simulink model "AFS_Model"  (R2021a)
settings: Solver=FixedStepDiscrete  StartTime=0.0  StopTime=1  FixedStep=0.2  RelTol=1e-3
libraries: simulink x25
settings Model: DataDictionary=AFLS.sldd  Creator=Prajakta  LastModifiedBy=hp
settings DataIOCC: ExternalInput=[t,Longi_Distance,Lat_Distance,Lux,Wheel_Angle,Speed]  LoadExternalInput=on
settings OptimizationCC: DefaultParameterBehavior=Inlined  EnhancedBackFolding=on  PassReuseOutputArgsAs=Individual arguments  ZeroExternalMemoryAtStartup=off  ZeroInternalMemoryAtStartup=off  OptimizeBlockOrder=speed  DifferentSizesBufferReuse=on  OptimizationCustomize=off  EfficientTunableParamExpr=on
settings DebuggingCC: ParameterTunabilityLossMsg=error
settings SFSimCC: MATLABDynamicMemAlloc=off
settings RTWCC: SystemTargetFile=ert.tlc  GenCodeOnly=on  TemplateMakefile=ert_default_tmf  GenerateReport=on  IncludeHyperlinkInReport=on  LaunchReport=on  GenerateTraceInfo=on  GenerateWebview=on
settings CodeAppCC: ForceParamTrailComments=on  IgnoreCustomStorageClasses=off  OperatorAnnotations=on  SimulinkDataObjDesc=on  SFDataObjDesc=on  InsertBlockDesc=on
settings ERTTargetCC: TargetLangStandard=C99 (ISO)  GenerateSampleERTMain=on  InlinedParameterPlacement=NonHierarchical  ERTCustomFileTemplate=example_file_process.tlc

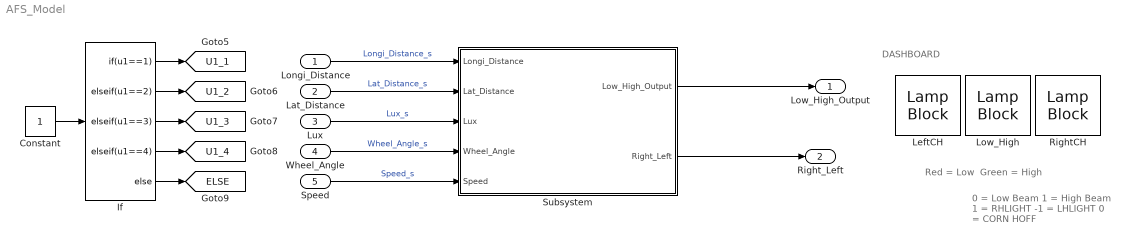
== system AFS_Model ==
  note: Green = High
  note: Red = Low
  note: 0 = Low Beam
      | 1 = High Beam
      | 1 = RHLIGHT
      | -1 = LHLIGHT
      | 0 = CORN HOFF
  note: DASHBOARD
  Longi_Distance : Inport
  Lat_Distance : Inport  Port=2
  Lux : Inport  Port=3
  Wheel_Angle : Inport  Port=4
  Speed : Inport  Port=5
  Constant : Constant
  If : If  IfExpression=u1==1  ElseIfExpressions=u1==2, u1==3,u1==4
  LeftCH : LampBlock
  Low_High : LampBlock
  RightCH : LampBlock
  Subsystem : Subsystem
  Low_High_Output : Outport
  Right_Left : Outport  Port=2
  tag scope: ELSE=global, U1_1=global, U1_2=global, U1_3=global, U1_4=global
  wires:
  If/1 -> [U1_1]
  If/2 -> [U1_2]
  If/3 -> [U1_3]
  If/4 -> [U1_4]
  If/5 -> [ELSE]
  Longi_Distance/1 -> Subsystem/1(Longi_Distance)  "Longi_Distance_s"
  Lat_Distance/1 -> Subsystem/2(Lat_Distance)  "Lat_Distance_s"
  Lux/1 -> Subsystem/3(Lux)  "Lux_s"
  Wheel_Angle/1 -> Subsystem/4(Wheel_Angle)  "Wheel_Angle_s"
  Speed/1 -> Subsystem/5(Speed)  "Speed_s"
  Subsystem/1(Low_High_Output) -> Low_High_Output/1
  Subsystem/2(Right_Left) -> Right_Left/1
  Constant/1 -> If/1

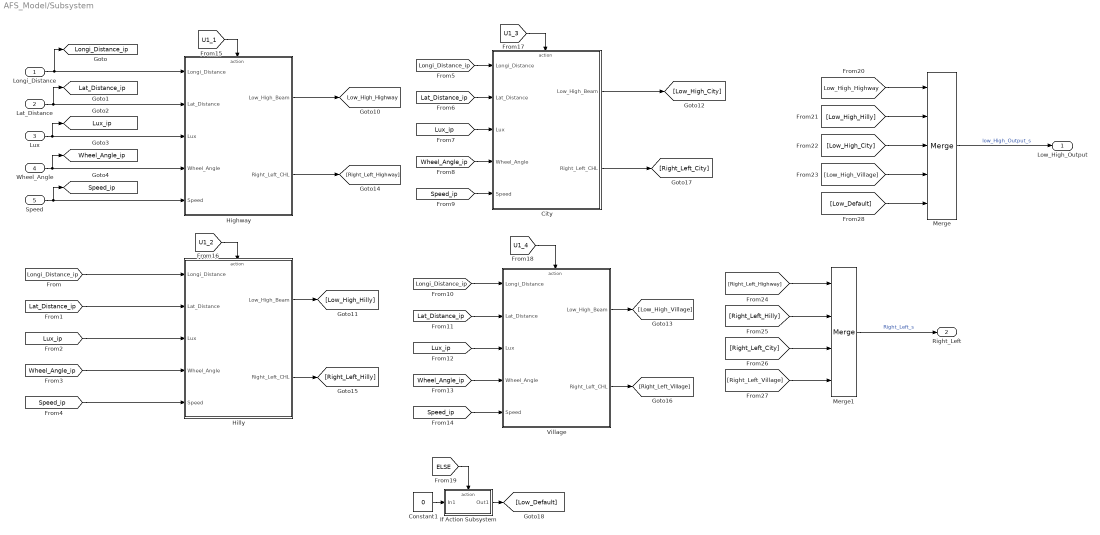
== system AFS_Model/Subsystem ==
  Longi_Distance : Inport
  Lat_Distance : Inport  Port=2
  Lux : Inport  Port=3
  Wheel_Angle : Inport  Port=4
  Speed : Inport  Port=5
  City : Subsystem  TreatAsAtomicUnit=on
  Constant1 : Constant  Value=0  OutDataTypeStr=int8
  Highway : Subsystem  TreatAsAtomicUnit=on
  Hilly : Subsystem  TreatAsAtomicUnit=on
  If Action Subsystem : Subsystem  TreatAsAtomicUnit=on
  Merge : Merge  Inputs=5
  Merge1 : Merge  Inputs=4
  Village : Subsystem  TreatAsAtomicUnit=on
  Low_High_Output : Outport
  Right_Left : Outport  Port=2  OutDataTypeStr=int8
  tag scope: Lat_Distance_ip=global, Longi_Distance_ip=global, Low_High_Highway=global, Lux_ip=global, Speed_ip=global, Wheel_Angle_ip=global
  wires:
  [ELSE] -> If Action Subsystem/Action
  [Wheel_Angle_ip] -> Hilly/4(Wheel_Angle)
  Longi_Distance/1 -> Highway/1(Longi_Distance), [Longi_Distance_ip]
  [Longi_Distance_ip] -> City/1(Longi_Distance)
  [Speed_ip] -> Hilly/5(Speed)
  [Low_High_Highway] -> Merge/1
  Lat_Distance/1 -> Highway/2(Lat_Distance), [Lat_Distance_ip]
  [Lux_ip] -> Hilly/3(Lux)
  [U1_2] -> Hilly/Action
  [U1_3] -> City/Action
  Wheel_Angle/1 -> Highway/4(Wheel_Angle), [Wheel_Angle_ip]
  [Low_Default] -> Merge/5
  City/2(Right_Left_CHL) -> [Right_Left_City]
  [Longi_Distance_ip] -> Hilly/1(Longi_Distance)
  Speed/1 -> Highway/5(Speed), [Speed_ip]
  [Wheel_Angle_ip] -> Village/4(Wheel_Angle)
  [Lat_Distance_ip] -> Hilly/2(Lat_Distance)
  [Lat_Distance_ip] -> City/2(Lat_Distance)
  Merge1/1 -> Right_Left/1  "Right_Left_s"
  Highway/2(Right_Left_CHL) -> [Right_Left_Highway]
  [Wheel_Angle_ip] -> City/4(Wheel_Angle)
  Highway/1(Low_High_Beam) -> [Low_High_Highway]
  Constant1/1 -> If Action Subsystem/1(In1)
  [U1_1] -> Highway/Action
  [Speed_ip] -> City/5(Speed)
  [Right_Left_Highway] -> Merge1/1
  [Longi_Distance_ip] -> Village/1(Longi_Distance)
  [U1_4] -> Village/Action
  Hilly/1(Low_High_Beam) -> [Low_High_Hilly]
  Lux/1 -> Highway/3(Lux), [Lux_ip]
  Hilly/2(Right_Left_CHL) -> [Right_Left_Hilly]
  Village/2(Right_Left_CHL) -> [Right_Left_Village]
  [Right_Left_Village] -> Merge1/4
  [Lux_ip] -> City/3(Lux)
  [Lat_Distance_ip] -> Village/2(Lat_Distance)
  [Right_Left_City] -> Merge1/3
  Village/1(Low_High_Beam) -> [Low_High_Village]
  [Speed_ip] -> Village/5(Speed)
  If Action Subsystem/1(Out1) -> [Low_Default]
  [Low_High_City] -> Merge/3
  [Lux_ip] -> Village/3(Lux)
  [Low_High_Village] -> Merge/4
  Merge/1 -> Low_High_Output/1  "low_High_Output_s"
  [Right_Left_Hilly] -> Merge1/2
  [Low_High_Hilly] -> Merge/2
  City/1(Low_High_Beam) -> [Low_High_City]

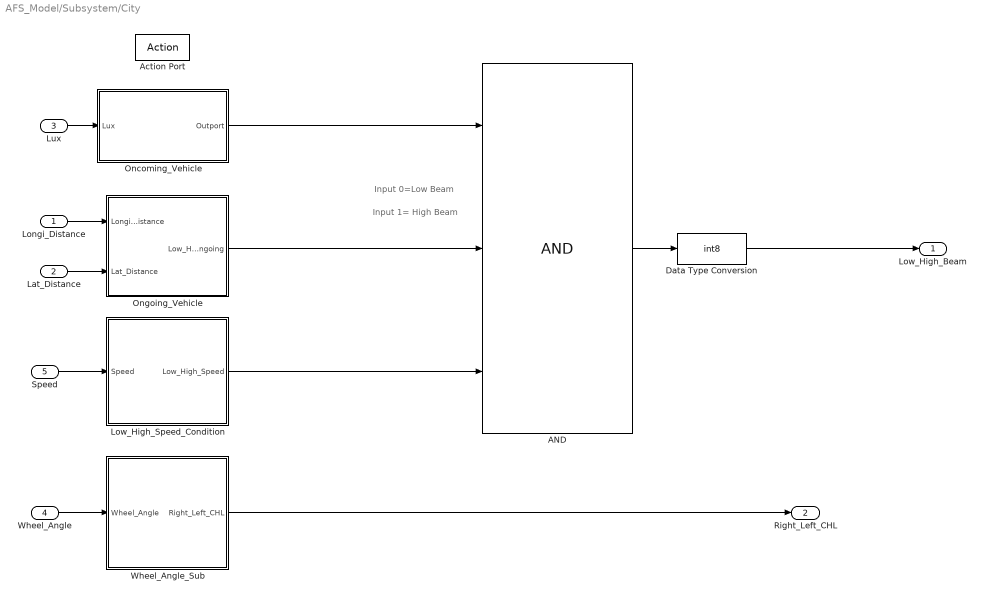
== system AFS_Model/Subsystem/City ==
  note: Input 1= High Beam
  note: Input 0=Low Beam
  Longi_Distance : Inport
  Lat_Distance : Inport  Port=2
  Lux : Inport  Port=3
  Wheel_Angle : Inport  Port=4
  Speed : Inport  Port=5
  Action Port : ActionPort  ActionPortLabel=elseif( u1==3)
  AND : Logic  Inputs=3  AllPortsSameDT=off  OutDataTypeStr=boolean
  Data Type Conversion : DataTypeConversion  OutDataTypeStr=int8
  Low_High_Speed_Condition : Subsystem
  Oncoming_Vehicle : Subsystem
  Ongoing_Vehicle : Subsystem
  Wheel_Angle_Sub : Subsystem
  Low_High_Beam : Outport
  Right_Left_CHL : Outport  Port=2
  wires:
  Longi_Distance/1 -> Ongoing_Vehicle/1(Longi_Distance)
  Lat_Distance/1 -> Ongoing_Vehicle/2(Lat_Distance)
  Lux/1 -> Oncoming_Vehicle/1(Lux)
  Oncoming_Vehicle/1(Outport) -> AND/1
  AND/1 -> Data Type Conversion/1
  Ongoing_Vehicle/1(Low_High_Ongoing) -> AND/2
  Data Type Conversion/1 -> Low_High_Beam/1
  Wheel_Angle/1 -> Wheel_Angle_Sub/1(Wheel_Angle)
  Wheel_Angle_Sub/1(Right_Left_CHL) -> Right_Left_CHL/1
  Low_High_Speed_Condition/1(Low_High_Speed) -> AND/3
  Speed/1 -> Low_High_Speed_Condition/1(Speed)

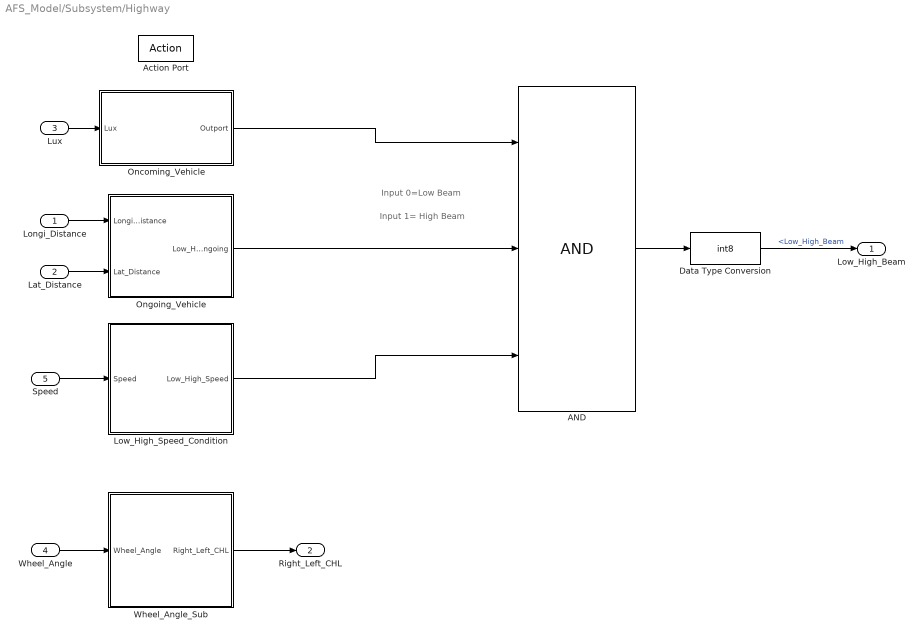
== system AFS_Model/Subsystem/Highway ==
  note: Input 1= High Beam
  note: Input 0=Low Beam
  Longi_Distance : Inport
  Lat_Distance : Inport  Port=2
  Lux : Inport  Port=3
  Wheel_Angle : Inport  Port=4
  Speed : Inport  Port=5
  Action Port : ActionPort  ActionPortLabel=if(u1==1)
  AND : Logic  Inputs=3  AllPortsSameDT=off  OutDataTypeStr=boolean
  Data Type Conversion : DataTypeConversion  OutDataTypeStr=int8
  Low_High_Speed_Condition : Subsystem
  Oncoming_Vehicle : Subsystem
  Ongoing_Vehicle : Subsystem
  Wheel_Angle_Sub : Subsystem
  Low_High_Beam : Outport
  Right_Left_CHL : Outport  Port=2
  wires:
  Longi_Distance/1 -> Ongoing_Vehicle/1(Longi_Distance)
  Lat_Distance/1 -> Ongoing_Vehicle/2(Lat_Distance)
  Lux/1 -> Oncoming_Vehicle/1(Lux)
  Oncoming_Vehicle/1(Outport) -> AND/1
  AND/1 -> Data Type Conversion/1
  Ongoing_Vehicle/1(Low_High_Ongoing) -> AND/2
  Data Type Conversion/1 -> Low_High_Beam/1  "<Low_High_Beam"
  Wheel_Angle/1 -> Wheel_Angle_Sub/1(Wheel_Angle)
  Wheel_Angle_Sub/1(Right_Left_CHL) -> Right_Left_CHL/1
  Low_High_Speed_Condition/1(Low_High_Speed) -> AND/3
  Speed/1 -> Low_High_Speed_Condition/1(Speed)

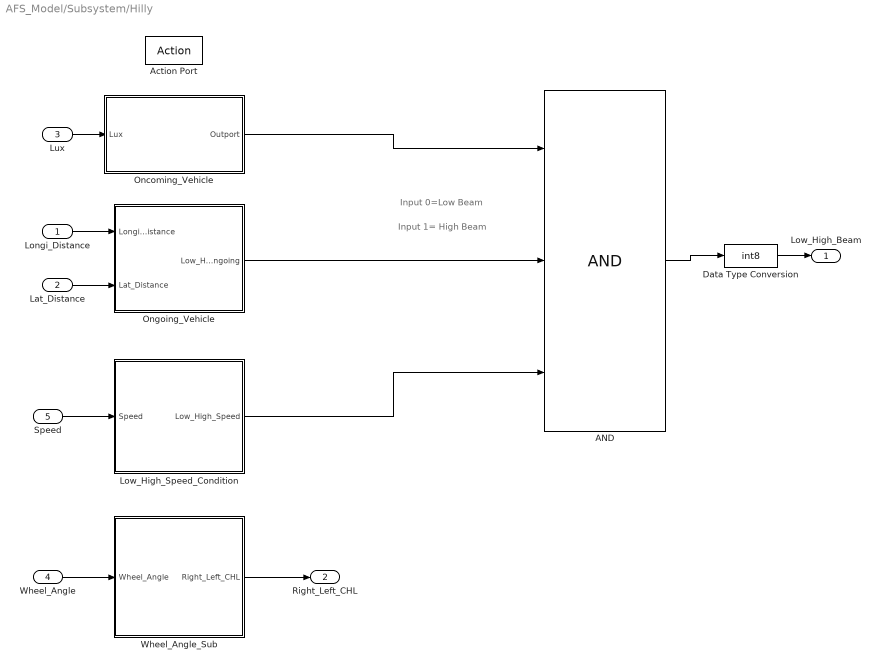
== system AFS_Model/Subsystem/Hilly ==
  note: Input 1= High Beam
  note: Input 0=Low Beam
  Longi_Distance : Inport
  Lat_Distance : Inport  Port=2
  Lux : Inport  Port=3
  Wheel_Angle : Inport  Port=4
  Speed : Inport  Port=5
  Action Port : ActionPort  ActionPortLabel=elseif(u1==2)
  AND : Logic  Inputs=3  AllPortsSameDT=off  OutDataTypeStr=boolean
  Data Type Conversion : DataTypeConversion  OutDataTypeStr=int8
  Low_High_Speed_Condition : Subsystem
  Oncoming_Vehicle : Subsystem
  Ongoing_Vehicle : Subsystem
  Wheel_Angle_Sub : Subsystem
  Low_High_Beam : Outport
  Right_Left_CHL : Outport  Port=2
  wires:
  Longi_Distance/1 -> Ongoing_Vehicle/1(Longi_Distance)
  Lat_Distance/1 -> Ongoing_Vehicle/2(Lat_Distance)
  Lux/1 -> Oncoming_Vehicle/1(Lux)
  Oncoming_Vehicle/1(Outport) -> AND/1
  AND/1 -> Data Type Conversion/1
  Ongoing_Vehicle/1(Low_High_Ongoing) -> AND/2
  Data Type Conversion/1 -> Low_High_Beam/1
  Wheel_Angle/1 -> Wheel_Angle_Sub/1(Wheel_Angle)
  Wheel_Angle_Sub/1(Right_Left_CHL) -> Right_Left_CHL/1
  Speed/1 -> Low_High_Speed_Condition/1(Speed)
  Low_High_Speed_Condition/1(Low_High_Speed) -> AND/3

== system AFS_Model/Subsystem/If Action Subsystem ==
  In1 : Inport  OutDataTypeStr=int8
  Action Port : ActionPort  ActionPortLabel=else
  Out1 : Outport  OutDataTypeStr=int8
  wires:
  In1/1 -> Out1/1

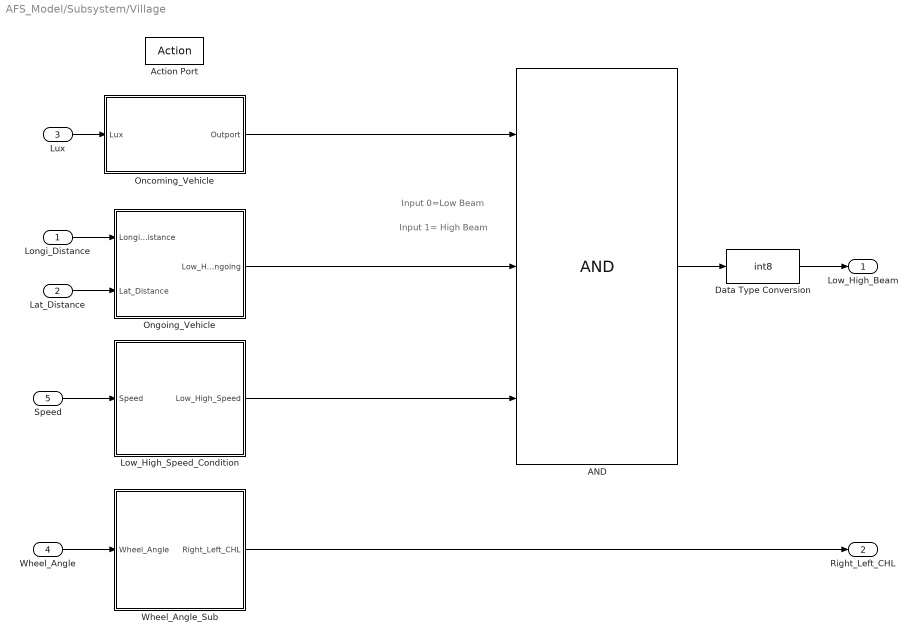
== system AFS_Model/Subsystem/Village ==
  note: Input 1= High Beam
  note: Input 0=Low Beam
  Longi_Distance : Inport
  Lat_Distance : Inport  Port=2
  Lux : Inport  Port=3
  Wheel_Angle : Inport  Port=4
  Speed : Inport  Port=5
  Action Port : ActionPort  ActionPortLabel=elseif(u1==4)
  AND : Logic  Inputs=3  AllPortsSameDT=off  OutDataTypeStr=boolean
  Data Type Conversion : DataTypeConversion  OutDataTypeStr=int8
  Low_High_Speed_Condition : Subsystem
  Oncoming_Vehicle : Subsystem
  Ongoing_Vehicle : Subsystem
  Wheel_Angle_Sub : Subsystem
  Low_High_Beam : Outport
  Right_Left_CHL : Outport  Port=2
  wires:
  Longi_Distance/1 -> Ongoing_Vehicle/1(Longi_Distance)
  Lat_Distance/1 -> Ongoing_Vehicle/2(Lat_Distance)
  Lux/1 -> Oncoming_Vehicle/1(Lux)
  Oncoming_Vehicle/1(Outport) -> AND/1
  AND/1 -> Data Type Conversion/1
  Ongoing_Vehicle/1(Low_High_Ongoing) -> AND/2
  Data Type Conversion/1 -> Low_High_Beam/1
  Wheel_Angle/1 -> Wheel_Angle_Sub/1(Wheel_Angle)
  Wheel_Angle_Sub/1(Right_Left_CHL) -> Right_Left_CHL/1
  Speed/1 -> Low_High_Speed_Condition/1(Speed)
  Low_High_Speed_Condition/1(Low_High_Speed) -> AND/3

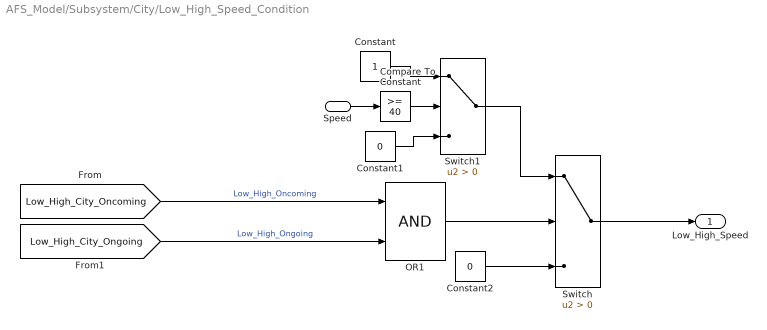
== system AFS_Model/Subsystem/City/Low_High_Speed_Condition ==
  Speed : Inport
  Compare To Constant : simulink/Logic and Bit Operations/Compare To Constant  relop=>=  const=40  OutDataTypeStr=boolean
  Constant : Constant  OutDataTypeStr=int8
  Constant1 : Constant  Value=0  OutDataTypeStr=int8
  Constant2 : Constant  Value=0  OutDataTypeStr=int8
  OR1 : Logic  AllPortsSameDT=off  OutDataTypeStr=boolean
  Switch : Switch  Criteria=u2 > Threshold  OutDataTypeStr=Inherit: Inherit via back propagation
  Switch1 : Switch  Criteria=u2 > Threshold
  Low_High_Speed : Outport  OutDataTypeStr=int8
  wires:
  [Low_High_City_Oncoming] -> OR1/1  "Low_High_Oncoming"
  [Low_High_City_Ongoing] -> OR1/2  "Low_High_Ongoing"
  Constant/1 -> Switch1/1
  Constant1/1 -> Switch1/3
  Compare To Constant/1 -> Switch1/2
  Switch/1 -> Low_High_Speed/1
  Speed/1 -> Compare To Constant/1
  Constant2/1 -> Switch/3
  Switch1/1 -> Switch/1
  OR1/1 -> Switch/2

== system AFS_Model/Subsystem/City/Oncoming_Vehicle ==
  note: ONCOMING VEHICAL LUX
  note: ONCOMING VEHICAL INPUTS AND OUTPUTS
  Lux : Inport
  Constant1 : Constant  Value=0  OutDataTypeStr=int8
  Constant2 : Constant  OutDataTypeStr=int8
  Switch : Switch  Threshold=20
  Outport : Outport  OutDataTypeStr=int8
  tag scope: Low_High_City_Oncoming=global
  wires:
  Lux/1 -> Switch/2
  Constant1/1 -> Switch/1
  Constant2/1 -> Switch/3
  Switch/1 -> [Low_High_City_Oncoming], Outport/1  "Low_High_Oncoming"

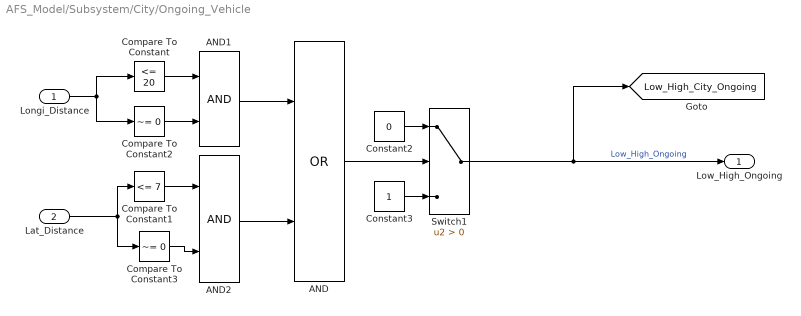
== system AFS_Model/Subsystem/City/Ongoing_Vehicle ==
  Longi_Distance : Inport
  Lat_Distance : Inport  Port=2
  AND : Logic  Operator=OR  AllPortsSameDT=off  OutDataTypeStr=boolean
  AND1 : Logic  AllPortsSameDT=off  OutDataTypeStr=boolean
  AND2 : Logic  AllPortsSameDT=off  OutDataTypeStr=boolean
  Compare To Constant : simulink/Logic and Bit Operations/Compare To Constant  relop=<=  const=20  OutDataTypeStr=boolean
  Compare To Constant1 : simulink/Logic and Bit Operations/Compare To Constant  relop=<=  const=7  OutDataTypeStr=boolean
  Compare To Constant2 : simulink/Logic and Bit Operations/Compare To Constant  relop=~=  const=0  OutDataTypeStr=boolean
  Compare To Constant3 : simulink/Logic and Bit Operations/Compare To Constant  relop=~=  const=0  OutDataTypeStr=boolean
  Constant2 : Constant  Value=0  OutDataTypeStr=int8
  Constant3 : Constant  OutDataTypeStr=int8
  Switch1 : Switch  Criteria=u2 > Threshold
  Low_High_Ongoing : Outport  OutDataTypeStr=int8
  tag scope: Low_High_City_Ongoing=global
  wires:
  Longi_Distance/1 -> Compare To Constant2/1, Compare To Constant/1
  Lat_Distance/1 -> Compare To Constant3/1, Compare To Constant1/1
  Compare To Constant1/1 -> AND2/1
  Compare To Constant/1 -> AND1/1
  Compare To Constant2/1 -> AND1/2
  AND1/1 -> AND/1
  Compare To Constant3/1 -> AND2/2
  AND2/1 -> AND/2
  Constant2/1 -> Switch1/1
  Constant3/1 -> Switch1/3
  Switch1/1 -> [Low_High_City_Ongoing], Low_High_Ongoing/1  "Low_High_Ongoing"
  AND/1 -> Switch1/2

== system AFS_Model/Subsystem/City/Wheel_Angle_Sub ==
  note: ANTI-CLOCKWISE DIRECTION
  note: VEHICAL WHEEL ANGLE INPUTS AND OUT-PUT
  note: CLOCKWISE DIRECTION
  note: DEFAULT CONDITION
  Wheel_Angle : Inport
  Compare To Constant : simulink/Logic and Bit Operations/Compare To Constant  relop=<=  const=-15  OutDataTypeStr=boolean
  Constant3 : Constant  OutDataTypeStr=int8
  Constant4 : Constant  Value=0  OutDataTypeStr=int8
  Constant5 : Constant  Value=-1  OutDataTypeStr=int8
  Switch : Switch  Threshold=15  OutDataTypeStr=Inherit: Inherit via back propagation
  Switch1 : Switch  Criteria=u2 > Threshold  OutDataTypeStr=Inherit: Inherit via back propagation
  Right_Left_CHL : Outport  OutDataTypeStr=int8
  wires:
  Wheel_Angle/1 -> Compare To Constant/1, Switch/2
  Constant3/1 -> Switch/1
  Compare To Constant/1 -> Switch1/2
  Constant5/1 -> Switch1/1
  Switch1/1 -> Switch/3
  Constant4/1 -> Switch1/3
  Switch/1 -> Right_Left_CHL/1

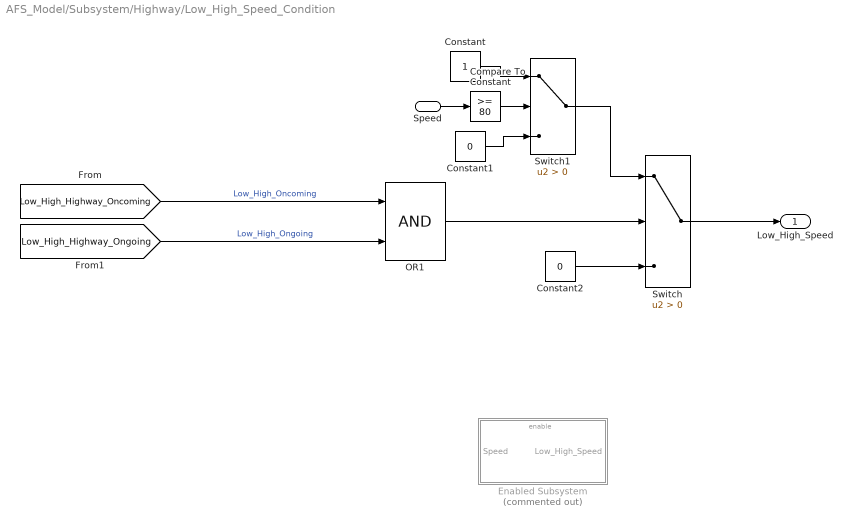
== system AFS_Model/Subsystem/Highway/Low_High_Speed_Condition ==
  Speed : Inport
  Compare To Constant : simulink/Logic and Bit Operations/Compare To Constant  relop=>=  const=80  OutDataTypeStr=boolean
  Constant : Constant  OutDataTypeStr=int8
  Constant1 : Constant  Value=0  OutDataTypeStr=int8
  Constant2 : Constant  Value=0  OutDataTypeStr=int8
  Enabled Subsystem : Subsystem  Commented=on  TreatAsAtomicUnit=on
  OR1 : Logic  AllPortsSameDT=off  OutDataTypeStr=boolean
  Switch : Switch  Criteria=u2 > Threshold  OutDataTypeStr=Inherit: Inherit via back propagation
  Switch1 : Switch  Criteria=u2 > Threshold
  Low_High_Speed : Outport  OutDataTypeStr=int8
  wires:
  [Low_High_Highway_Oncoming] -> OR1/1  "Low_High_Oncoming"
  [Low_High_Highway_Ongoing] -> OR1/2  "Low_High_Ongoing"
  Switch/1 -> Low_High_Speed/1
  Constant2/1 -> Switch/3
  Speed/1 -> Compare To Constant/1
  Compare To Constant/1 -> Switch1/2
  OR1/1 -> Switch/2
  Switch1/1 -> Switch/1
  Constant/1 -> Switch1/1
  Constant1/1 -> Switch1/3

== system AFS_Model/Subsystem/Highway/Oncoming_Vehicle ==
  note: ONCOMING VEHICAL LUX
  note: ONCOMING VEHICAL INPUTS AND OUTPUTS
  Lux : Inport
  Constant1 : Constant  Value=0  OutDataTypeStr=int8
  Constant2 : Constant  OutDataTypeStr=int8
  Switch : Switch  Threshold=20
  Outport : Outport  OutDataTypeStr=int8
  tag scope: Low_High_Highway_Oncoming=global
  wires:
  Lux/1 -> Switch/2
  Constant1/1 -> Switch/1
  Constant2/1 -> Switch/3
  Switch/1 -> [Low_High_Highway_Oncoming], Outport/1  "Low_High_Oncoming"

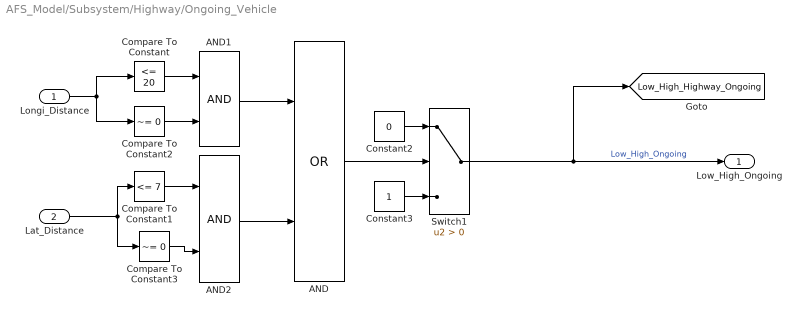
== system AFS_Model/Subsystem/Highway/Ongoing_Vehicle ==
  Longi_Distance : Inport
  Lat_Distance : Inport  Port=2
  AND : Logic  Operator=OR  AllPortsSameDT=off  OutDataTypeStr=boolean
  AND1 : Logic  AllPortsSameDT=off  OutDataTypeStr=boolean
  AND2 : Logic  AllPortsSameDT=off  OutDataTypeStr=boolean
  Compare To Constant : simulink/Logic and Bit Operations/Compare To Constant  relop=<=  const=20  OutDataTypeStr=boolean
  Compare To Constant1 : simulink/Logic and Bit Operations/Compare To Constant  relop=<=  const=7  OutDataTypeStr=boolean
  Compare To Constant2 : simulink/Logic and Bit Operations/Compare To Constant  relop=~=  const=0  OutDataTypeStr=boolean
  Compare To Constant3 : simulink/Logic and Bit Operations/Compare To Constant  relop=~=  const=0  OutDataTypeStr=boolean
  Constant2 : Constant  Value=0  OutDataTypeStr=int8
  Constant3 : Constant  OutDataTypeStr=int8
  Switch1 : Switch  Criteria=u2 > Threshold
  Low_High_Ongoing : Outport  OutDataTypeStr=int8
  tag scope: Low_High_Highway_Ongoing=global
  wires:
  Longi_Distance/1 -> Compare To Constant2/1, Compare To Constant/1
  Lat_Distance/1 -> Compare To Constant3/1, Compare To Constant1/1
  Compare To Constant1/1 -> AND2/1
  Compare To Constant/1 -> AND1/1
  Compare To Constant2/1 -> AND1/2
  AND1/1 -> AND/1
  Compare To Constant3/1 -> AND2/2
  AND2/1 -> AND/2
  Constant2/1 -> Switch1/1
  Constant3/1 -> Switch1/3
  Switch1/1 -> [Low_High_Highway_Ongoing], Low_High_Ongoing/1  "Low_High_Ongoing"
  AND/1 -> Switch1/2

== system AFS_Model/Subsystem/Highway/Wheel_Angle_Sub ==
  note: ANTI-CLOCKWISE DIRECTION
  note: VEHICAL WHEEL ANGLE INPUTS AND OUT-PUT
  note: CLOCKWISE DIRECTION
  note: DEFAULT CONDITION
  Wheel_Angle : Inport
  Compare To Constant : simulink/Logic and Bit Operations/Compare To Constant  relop=<=  const=-15  OutDataTypeStr=boolean
  Constant3 : Constant  OutDataTypeStr=int8
  Constant4 : Constant  Value=0  OutDataTypeStr=int8
  Constant5 : Constant  Value=-1  OutDataTypeStr=int8
  Switch : Switch  Threshold=15  OutDataTypeStr=Inherit: Inherit via back propagation
  Switch1 : Switch  Criteria=u2 > Threshold  OutDataTypeStr=Inherit: Inherit via back propagation
  Right_Left_CHL : Outport  OutDataTypeStr=int8
  wires:
  Wheel_Angle/1 -> Compare To Constant/1, Switch/2
  Constant3/1 -> Switch/1
  Compare To Constant/1 -> Switch1/2
  Constant5/1 -> Switch1/1
  Switch1/1 -> Switch/3
  Constant4/1 -> Switch1/3
  Switch/1 -> Right_Left_CHL/1

== system AFS_Model/Subsystem/Hilly/Low_High_Speed_Condition ==
  Speed : Inport
  Compare To Constant : simulink/Logic and Bit Operations/Compare To Constant  relop=>=  const=60  OutDataTypeStr=boolean
  Constant : Constant  OutDataTypeStr=int8
  Constant1 : Constant  Value=0  OutDataTypeStr=int8
  Constant2 : Constant  Value=0  OutDataTypeStr=int8
  OR1 : Logic  AllPortsSameDT=off  OutDataTypeStr=boolean
  Switch : Switch  Criteria=u2 > Threshold  OutDataTypeStr=Inherit: Inherit via back propagation
  Switch1 : Switch  Criteria=u2 > Threshold
  Low_High_Speed : Outport  OutDataTypeStr=int8
  wires:
  [Low_High_Hilly_Oncoming] -> OR1/1  "Low_High_Oncoming"
  [Low_High_Hilly_Ongoing] -> OR1/2  "Low_High_Ongoing"
  Constant/1 -> Switch1/1
  Constant1/1 -> Switch1/3
  Compare To Constant/1 -> Switch1/2
  Switch/1 -> Low_High_Speed/1
  Speed/1 -> Compare To Constant/1
  Constant2/1 -> Switch/3
  Switch1/1 -> Switch/1
  OR1/1 -> Switch/2

== system AFS_Model/Subsystem/Hilly/Oncoming_Vehicle ==
  note: ONCOMING VEHICAL LUX
  note: ONCOMING VEHICAL INPUTS AND OUTPUTS
  Lux : Inport
  Constant1 : Constant  Value=0  OutDataTypeStr=int8
  Constant2 : Constant  OutDataTypeStr=int8
  Switch : Switch  Threshold=20
  Outport : Outport  OutDataTypeStr=int8
  tag scope: Low_High_Hilly_Oncoming=global
  wires:
  Lux/1 -> Switch/2
  Constant1/1 -> Switch/1
  Constant2/1 -> Switch/3
  Switch/1 -> [Low_High_Hilly_Oncoming], Outport/1  "Low_High_Oncoming"

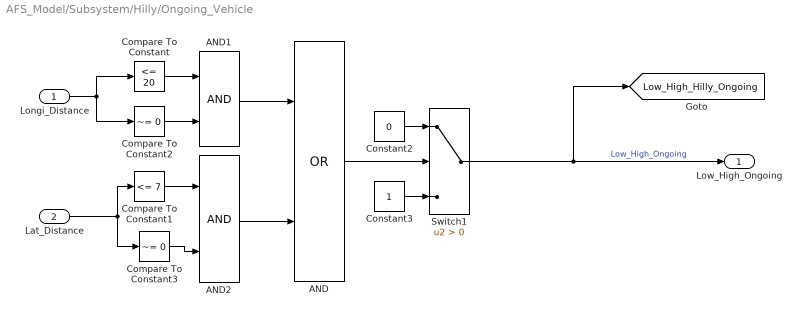
== system AFS_Model/Subsystem/Hilly/Ongoing_Vehicle ==
  Longi_Distance : Inport
  Lat_Distance : Inport  Port=2
  AND : Logic  Operator=OR  AllPortsSameDT=off  OutDataTypeStr=boolean
  AND1 : Logic  AllPortsSameDT=off  OutDataTypeStr=boolean
  AND2 : Logic  AllPortsSameDT=off  OutDataTypeStr=boolean
  Compare To Constant : simulink/Logic and Bit Operations/Compare To Constant  relop=<=  const=20  OutDataTypeStr=boolean
  Compare To Constant1 : simulink/Logic and Bit Operations/Compare To Constant  relop=<=  const=7  OutDataTypeStr=boolean
  Compare To Constant2 : simulink/Logic and Bit Operations/Compare To Constant  relop=~=  const=0  OutDataTypeStr=boolean
  Compare To Constant3 : simulink/Logic and Bit Operations/Compare To Constant  relop=~=  const=0  OutDataTypeStr=boolean
  Constant2 : Constant  Value=0  OutDataTypeStr=int8
  Constant3 : Constant  OutDataTypeStr=int8
  Switch1 : Switch  Criteria=u2 > Threshold
  Low_High_Ongoing : Outport  OutDataTypeStr=int8
  tag scope: Low_High_Hilly_Ongoing=global
  wires:
  Longi_Distance/1 -> Compare To Constant2/1, Compare To Constant/1
  Lat_Distance/1 -> Compare To Constant3/1, Compare To Constant1/1
  Compare To Constant1/1 -> AND2/1
  Compare To Constant/1 -> AND1/1
  Compare To Constant2/1 -> AND1/2
  AND1/1 -> AND/1
  Compare To Constant3/1 -> AND2/2
  AND2/1 -> AND/2
  Constant2/1 -> Switch1/1
  Constant3/1 -> Switch1/3
  Switch1/1 -> [Low_High_Hilly_Ongoing], Low_High_Ongoing/1  "Low_High_Ongoing"
  AND/1 -> Switch1/2

== system AFS_Model/Subsystem/Hilly/Wheel_Angle_Sub ==
  note: ANTI-CLOCKWISE DIRECTION
  note: VEHICAL WHEEL ANGLE INPUTS AND OUT-PUT
  note: CLOCKWISE DIRECTION
  note: DEFAULT CONDITION
  Wheel_Angle : Inport
  Compare To Constant : simulink/Logic and Bit Operations/Compare To Constant  relop=<=  const=-15  OutDataTypeStr=boolean
  Constant3 : Constant  OutDataTypeStr=int8
  Constant4 : Constant  Value=0  OutDataTypeStr=int8
  Constant5 : Constant  Value=-1  OutDataTypeStr=int8
  Switch : Switch  Threshold=15  OutDataTypeStr=Inherit: Inherit via back propagation
  Switch1 : Switch  Criteria=u2 > Threshold  OutDataTypeStr=Inherit: Inherit via back propagation
  Right_Left_CHL : Outport  OutDataTypeStr=int8
  wires:
  Wheel_Angle/1 -> Compare To Constant/1, Switch/2
  Constant3/1 -> Switch/1
  Compare To Constant/1 -> Switch1/2
  Constant5/1 -> Switch1/1
  Switch1/1 -> Switch/3
  Constant4/1 -> Switch1/3
  Switch/1 -> Right_Left_CHL/1

== system AFS_Model/Subsystem/Village/Low_High_Speed_Condition ==
  Speed : Inport
  Compare To Constant : simulink/Logic and Bit Operations/Compare To Constant  relop=>=  const=20  OutDataTypeStr=boolean
  Constant : Constant  OutDataTypeStr=int8
  Constant1 : Constant  Value=0  OutDataTypeStr=int8
  Constant2 : Constant  Value=0  OutDataTypeStr=int8
  OR1 : Logic  AllPortsSameDT=off  OutDataTypeStr=boolean
  Switch : Switch  Criteria=u2 > Threshold  OutDataTypeStr=Inherit: Inherit via back propagation
  Switch1 : Switch  Criteria=u2 > Threshold
  Low_High_Speed : Outport  OutDataTypeStr=int8
  wires:
  [Low_High_Village_Oncoming] -> OR1/1  "Low_High_Oncoming"
  [Low_High_Village_Ongoing] -> OR1/2  "Low_High_Ongoing"
  Constant/1 -> Switch1/1
  Constant1/1 -> Switch1/3
  Compare To Constant/1 -> Switch1/2
  Switch/1 -> Low_High_Speed/1
  Speed/1 -> Compare To Constant/1
  Constant2/1 -> Switch/3
  Switch1/1 -> Switch/1
  OR1/1 -> Switch/2

== system AFS_Model/Subsystem/Village/Oncoming_Vehicle ==
  note: ONCOMING VEHICAL LUX
  note: ONCOMING VEHICAL INPUTS AND OUTPUTS
  Lux : Inport
  Constant1 : Constant  Value=0  OutDataTypeStr=int8
  Constant2 : Constant  OutDataTypeStr=int8
  Signal Conversion : SignalConversion  OverrideOpt=off
  Switch : Switch  Threshold=20
  Outport : Outport  OutDataTypeStr=int8
  tag scope: Low_High_Village_Oncoming=global
  wires:
  Lux/1 -> Switch/2
  Constant1/1 -> Switch/1
  Constant2/1 -> Switch/3
  Switch/1 -> Signal Conversion/1
  Signal Conversion/1 -> [Low_High_Village_Oncoming], Outport/1  "Low_High_Oncoming"

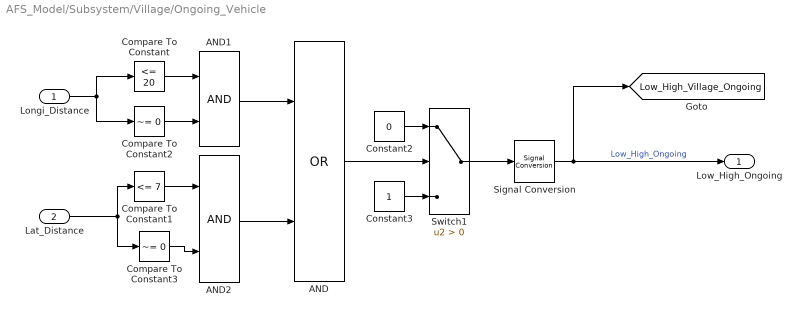
== system AFS_Model/Subsystem/Village/Ongoing_Vehicle ==
  Longi_Distance : Inport
  Lat_Distance : Inport  Port=2
  AND : Logic  Operator=OR  AllPortsSameDT=off  OutDataTypeStr=boolean
  AND1 : Logic  AllPortsSameDT=off  OutDataTypeStr=boolean
  AND2 : Logic  AllPortsSameDT=off  OutDataTypeStr=boolean
  Compare To Constant : simulink/Logic and Bit Operations/Compare To Constant  relop=<=  const=20  OutDataTypeStr=boolean
  Compare To Constant1 : simulink/Logic and Bit Operations/Compare To Constant  relop=<=  const=7  OutDataTypeStr=boolean
  Compare To Constant2 : simulink/Logic and Bit Operations/Compare To Constant  relop=~=  const=0  OutDataTypeStr=boolean
  Compare To Constant3 : simulink/Logic and Bit Operations/Compare To Constant  relop=~=  const=0  OutDataTypeStr=boolean
  Constant2 : Constant  Value=0  OutDataTypeStr=int8
  Constant3 : Constant  OutDataTypeStr=int8
  Signal Conversion : SignalConversion  OverrideOpt=off
  Switch1 : Switch  Criteria=u2 > Threshold
  Low_High_Ongoing : Outport  OutDataTypeStr=int8
  tag scope: Low_High_Village_Ongoing=global
  wires:
  Longi_Distance/1 -> Compare To Constant2/1, Compare To Constant/1
  Lat_Distance/1 -> Compare To Constant3/1, Compare To Constant1/1
  Compare To Constant1/1 -> AND2/1
  Compare To Constant/1 -> AND1/1
  Compare To Constant2/1 -> AND1/2
  AND1/1 -> AND/1
  Compare To Constant3/1 -> AND2/2
  AND2/1 -> AND/2
  Switch1/1 -> Signal Conversion/1
  Constant2/1 -> Switch1/1
  Constant3/1 -> Switch1/3
  Signal Conversion/1 -> [Low_High_Village_Ongoing], Low_High_Ongoing/1  "Low_High_Ongoing"
  AND/1 -> Switch1/2

== system AFS_Model/Subsystem/Village/Wheel_Angle_Sub ==
  note: ANTI-CLOCKWISE DIRECTION
  note: VEHICAL WHEEL ANGLE INPUTS AND OUT-PUT
  note: CLOCKWISE DIRECTION
  note: DEFAULT CONDITION
  Wheel_Angle : Inport
  Compare To Constant : simulink/Logic and Bit Operations/Compare To Constant  relop=<=  const=-15  OutDataTypeStr=boolean
  Constant3 : Constant  OutDataTypeStr=int8
  Constant4 : Constant  Value=0  OutDataTypeStr=int8
  Constant5 : Constant  Value=-1  OutDataTypeStr=int8
  Switch : Switch  Threshold=15  OutDataTypeStr=Inherit: Inherit via back propagation
  Switch1 : Switch  Criteria=u2 > Threshold  OutDataTypeStr=Inherit: Inherit via back propagation
  Right_Left_CHL : Outport  OutDataTypeStr=int8
  wires:
  Wheel_Angle/1 -> Compare To Constant/1, Switch/2
  Constant3/1 -> Switch/1
  Compare To Constant/1 -> Switch1/2
  Constant5/1 -> Switch1/1
  Switch1/1 -> Switch/3
  Constant4/1 -> Switch1/3
  Switch/1 -> Right_Left_CHL/1

== system AFS_Model/Subsystem/Highway/Low_High_Speed_Condition/Enabled Subsystem ==
  Speed : Inport
  Enable : EnablePort
  Compare To Constant : simulink/Logic and Bit Operations/Compare To Constant  relop=>=  const=80  OutDataTypeStr=boolean
  Constant : Constant
  Constant2 : Constant  Value=0
  Switch : Switch  Criteria=u2 > Threshold
  Low_High_Speed : Outport
  wires:
  Compare To Constant/1 -> Switch/2
  Speed/1 -> Compare To Constant/1
  Constant/1 -> Switch/1
  Constant2/1 -> Switch/3
  Switch/1 -> Low_High_Speed/1
